simulink library "AE511Library"  (R2018b)
settings: Solver=VariableStepAuto  StartTime=0.0  StopTime=10.0  RelTol=1e-3
settings Model: Creator=Christopher  LastModifiedBy=Christopher

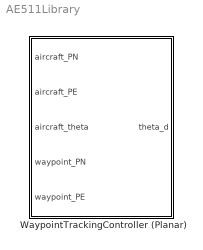
== system AE511Library ==
  WaypointTrackingController (Planar) : Subsystem
      mask help:
      | Determine the heading angle the aircraft should have in order to be pointing towards the waypoint.
      |
      | PARAMETERS:
      | -None
      |
      | INPUT:
      | -aircraft_PN: position north of the aircraft
      | -aircraft_PE: position east of the aircraft
      | -aircraft_theta: heading angle of the aircraft (0 = pointing East, positive CCW)
      | -waypoint_PN: position north of the waypoint
      | -waypoint_PE: position east of the waypoint
      |
      | OUTPUT:
      | -theta_d: desired heading angle so aircraft is pointing towards waypoint
      |
      | Created by Christopher Lum
      | lum@uw.edu

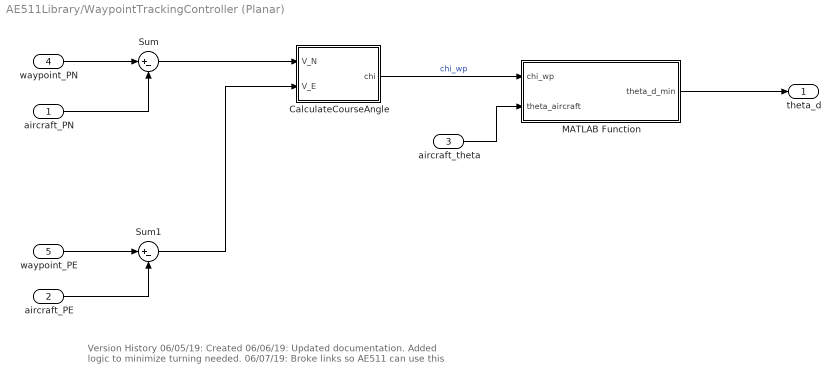
== system AE511Library/WaypointTrackingController (Planar) ==
  note: Version History
      | 06/05/19: Created
      | 06/06/19: Updated documentation.  Added logic to minimize turning needed.
      | 06/07/19: Broke links so AE511 can use this
  aircraft_PN : Inport
  aircraft_PE : Inport  Port=2
  aircraft_theta : Inport  Port=3
  waypoint_PN : Inport  Port=4
  waypoint_PE : Inport  Port=5
  CalculateCourseAngle : Subsystem
      mask help:
      | Calculate the course angle (chie) given the north velocity (V_N) and east velocity (V_E).
      |
      | A heading of chi = 0 implies a course of directly north.
      |
      | The units of V_N and V_E must be teh same.  chi is restricted to the range of [0, 2*pi).
      |
      | INPUTS:
      | -V_N: North velocity
      | -V_E: East velocity
      |
      | OUTPUTS:
      | -chi: course angle in range of [0, 2*pi) (radians)
      |
      | Created by Christopher Lum
      | lum@uw.edu
  MATLAB Function : MATLAB Function  TreatAsAtomicUnit=on
  Sum : Sum  Inputs=|+-
  Sum1 : Sum  Inputs=|+-
  theta_d : Outport
  wires:
  waypoint_PN/1 -> Sum/1
  aircraft_PN/1 -> Sum/2
  waypoint_PE/1 -> Sum1/1
  aircraft_PE/1 -> Sum1/2
  Sum/1 -> CalculateCourseAngle/1(V_N)
  Sum1/1 -> CalculateCourseAngle/2(V_E)
  CalculateCourseAngle/1(chi) -> MATLAB Function/1(chi_wp)  "chi_wp"
  aircraft_theta/1 -> MATLAB Function/2(theta_aircraft)
  MATLAB Function/1(theta_d_min) -> theta_d/1

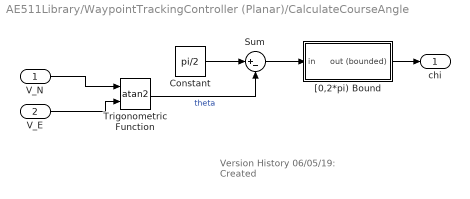
== system AE511Library/WaypointTrackingController (Planar)/CalculateCourseAngle ==
  note: Version History
      | 06/05/19: Created
  V_N : Inport
  V_E : Inport  Port=2
  Constant : Constant  Value=pi/2
  Sum : Sum  Inputs=|+-
  Trigonometric Function : Trigonometry  Operator=atan2
  "[0,2*pi) Bound" : Subsystem  Description=|
      | Version History  
      |                  
      | 05/??/05: Created
      mask help:
      | Converts input angle to it equivalent in the range [0,2*pi).
      |
      | Inputs:		In: input angle (rad)
      | Outputs:	Out (bounded): bounded angle in range [0,2*pi).
      |
      | Created by Christopher Lum
      | lum@u.washington.edu
      |
      | Original Block concept from Aerosim Blockset by Unmanned Dynamics.  www.u-dynamics.com
  chi : Outport
  wires:
  Sum/1 -> "[0,2*pi) Bound"/1(in)
  Constant/1 -> Sum/1
  Trigonometric Function/1 -> Sum/2  "theta"
  "[0,2*pi) Bound"/1(out (bounded)) -> chi/1
  V_E/1 -> Trigonometric Function/2
  V_N/1 -> Trigonometric Function/1

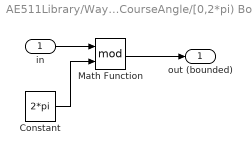
== system AE511Library/WaypointTrackingController (Planar)/CalculateCourseAngle/[0,2*pi) Bound ==
  in : Inport
  Constant : Constant  Value=2*pi
  Math Function : Math  Operator=mod  SaturateOnIntegerOverflow=on
  out (bounded) : Outport
  wires:
  in/1 -> Math Function/1
  Math Function/1 -> out (bounded)/1
  Constant/1 -> Math Function/2

== matlab function AE511Library/WaypointTrackingController (Planar)/MATLAB Function ==
  data: chi_wp input; theta_d_min output; theta_aircraft input
function theta_d_min  = fcn(chi_wp, theta_aircraft)

%convert chi to theta
theta_d = pi/2 - chi_wp;

%Determine if we need to add or subtract 2*pi to minimize required turning
theta_d_p2p = theta_d + 2*pi;
theta_d_m2p = theta_d - 2*pi;

%which yields the least error between the current aircraft theta
e_theta = theta_d - theta_aircraft;
e_theta_p2p = theta_d_p2p - theta_aircraft;
e_theta_m2p = theta_d_m2p - theta_aircraft;

[~,index] = min(abs([e_theta e_theta_p2p e_theta_m2p]));

switch index
    case 1
        %theta_d is best
        theta_d_min = theta_d;
        
    case 2
        %theta_d_p2p is best
        theta_d_min = theta_d_p2p;
        
    case 3
        %theta_d_m2p is best
        theta_d_min = e_theta_m2p;
        
    otherwise
        error('Unexpected error')
end
